simulink model "GFL_phasejump"  (R2022a)
settings: Solver=FixedStepAuto  StartTime=0.0  StopTime=t_end+t_sim_start  FixedStep=Ts  RelTol=1e-3
undefined symbols (not defined in the file or in its folder): Cf, dc_ref, DiscIntNeverNeededParam, dt, Id0, Id_limit, initial, Iq0, ki_pll, ki_v_dc, kp_pll, kp_v_dc, Lc, Lf, Lg1, Lg11, Lgg, m_v, phasejum, Rf, Rg1, Rg11, Rgg, Sbase, t0, t0_jump, t_sim_start, tc, Ts, v_sag, Vac_ref, Vbase, Vdc_ref, w_i_GFL, w_limit, w_pll, w_tau, w_tvc, Wbase, Y_dc, Zbase
libraries: spsVoltageMeasurementLib x41, spsCurrentMeasurementLib x36, spsThreePhaseSeriesRLCBranchLib x14, spsControlledVoltageSourceLib x12, spsSeriesRLCBranchLib x8, spsControlledCurrentSourceLib x4, spsIdealSwitchLib x3, spsThreePhaseBreakerLib x2, spsDCVoltageSourceLib x1, spsThreePhaseParallelRLCBranchLib x1, spsThreePhaseFaultLib x1, spspowerguiLib x1
(part 3 of 3)

== system GFL_phasejump/Grid-Following Inverter (Simulink Block)1/PLL (vabc -> vq)/Discrete PI ==
  note: Digital PI controller
      |
      | Author(s): Yitong Li
  enable : Inport
  reference : Inport  Port=2
  initial : Inport  Port=3
  actual : Inport  Port=4
  Discrete-Time Integrator : DiscreteIntegrator  gainval=1  ExternalReset=rising  InitialConditionSource=external  InitialCondition=initial  SampleTime=Ts  LimitOutput=on  UpperSaturationLimit=xmax  LowerSaturationLimit=xmin  ICPrevOutput=DiscIntNeverNeededParam  ICPrevScaledInput=DiscIntNeverNeededParam
  Ierror : Sum  Inputs=+-
  Ki : Gain  Gain=Ki  SaturateOnIntegerOverflow=on  OutDataTypeStr=Inherit: Same as input  ParamDataTypeStr=Inherit: Same as input
  Kp : Gain  Gain=Kp  SaturateOnIntegerOverflow=on  OutDataTypeStr=Inherit: Same as input  ParamDataTypeStr=Inherit: Same as input
  Perror : Sum  Inputs=-+
  Product : Product  RndMeth=Zero
  Product1 : Product  RndMeth=Zero
  Saturation : Saturate  UpperLimit=xmax  LowerLimit=xmin
  Scope : Scope  NumInputPorts=4
  Sum1 : Sum  SaturateOnIntegerOverflow=on
  Out : Outport
  wires:
  Product1/1 -> Ki/1
  Ierror/1 -> Product1/1
  Product/1 -> Kp/1
  Perror/1 -> Product/1
  actual/1 -> Perror/1, Ierror/2
  reference/1 -> Ierror/1, Perror/2
  initial/1 -> Discrete-Time Integrator/3
  enable/1 -> Product1/2, Product/2, Discrete-Time Integrator/2
  Discrete-Time Integrator/1 -> Scope/2, Sum1/2
  Kp/1 -> Scope/1, Sum1/1
  Ki/1 -> Discrete-Time Integrator/1
  Sum1/1 -> Saturation/1
  Saturation/1 -> Out/1

== system GFL_phasejump/Grid-Following Inverter (Simulink Block)1/PLL (vabc -> vq)/abc -> dq (Power-Invariant) ==
  note: Frame transformation from abc to dq.
      |
      | Author(s): Yitong Li
      |
      | Notes:
      |
      | The transformation is power-invariant.
      |
      | theta is the angle that d axis leads a axis.
      |
      | q axis leads d axis by 90 degrees.
  abc : Inport
  theta : Inport  Port=2
  ->d : Fcn  Expr=cos(u(4))*u(1) + cos(u(4)-2/3*pi)*u(2) + cos(u(4)-4/3*pi)*u(3)
  ->q : Fcn  Expr=-sin(u(4))*u(1) - sin(u(4)-2/3*pi)*u(2) - sin(u(4)-4/3*pi)*u(3)
  Gain : Gain  Gain=sqrt(2/3)
  Mux5 : Mux  Inputs=2
  Mux6 : Mux  Inputs=2
  dq : Outport
  wires:
  abc/1 -> Gain/1
  ->d/1 -> Mux6/1
  Gain/1 -> Mux5/1
  theta/1 -> Mux5/2
  ->q/1 -> Mux6/2
  Mux6/1 -> dq/1
  Mux5/1 -> ->d/1, ->q/1

== system GFL_phasejump/Grid-Following Inverter (Simulink Block)1/Voltage Controller/PI-DT-Estimated q ==
  actual : Inport
  initial : Inport  Port=2
  reference : Inport  Port=3
  enable : Inport  Port=4
  Discrete-Time Integrator : DiscreteIntegrator  gainval=1  ExternalReset=rising  InitialCondition=1  SampleTime=Ts  LimitOutput=on  UpperSaturationLimit=xmax  LowerSaturationLimit=xmin  ICPrevOutput=DiscIntNeverNeededParam  ICPrevScaledInput=DiscIntNeverNeededParam
  Ierror : Sum  Inputs=+-
  Ki : Gain  Gain=Ki  SaturateOnIntegerOverflow=on  OutDataTypeStr=Inherit: Same as input  ParamDataTypeStr=Inherit: Same as input
  Kp : Gain  Gain=Kp  SaturateOnIntegerOverflow=on  OutDataTypeStr=Inherit: Same as input  ParamDataTypeStr=Inherit: Same as input
  Perror : Sum  Inputs=-+
  Product : Product  RndMeth=Zero
  Product1 : Product  RndMeth=Zero
  Saturation : Saturate  UpperLimit=xmax  LowerLimit=xmin
  Sum1 : Sum  SaturateOnIntegerOverflow=on
  Out : Outport
  wires:
  Product1/1 -> Ki/1
  Ierror/1 -> Product1/1
  Product/1 -> Kp/1
  Perror/1 -> Product/1
  enable/1 -> Product1/2, Product/2, Discrete-Time Integrator/2
  Discrete-Time Integrator/1 -> Sum1/2
  Kp/1 -> Sum1/1
  Ki/1 -> Discrete-Time Integrator/1
  Sum1/1 -> Saturation/1
  Saturation/1 -> Out/1
  actual/1 -> Ierror/1, Perror/2
  reference/1 -> Ierror/2, Perror/1

== system GFL_phasejump/Grid-Following Inverter (Simulink Block)2/Current Controller/PI-DT-Estimated d ==
  enable : Inport
  reference : Inport  Port=2
  initial : Inport  Port=3
  actual : Inport  Port=4
  Discrete-Time Integrator : DiscreteIntegrator  gainval=1  ExternalReset=rising  InitialConditionSource=external  InitialCondition=initial  SampleTime=Ts  LimitOutput=on  UpperSaturationLimit=xmax  LowerSaturationLimit=xmin  ICPrevOutput=DiscIntNeverNeededParam  ICPrevScaledInput=DiscIntNeverNeededParam
  Ierror : Sum  Inputs=+-
  Ki : Gain  Gain=Ki  SaturateOnIntegerOverflow=on  OutDataTypeStr=Inherit: Same as input  ParamDataTypeStr=Inherit: Same as input
  Kp : Gain  Gain=Kp  SaturateOnIntegerOverflow=on  OutDataTypeStr=Inherit: Same as input  ParamDataTypeStr=Inherit: Same as input
  Perror : Sum  Inputs=-+
  Product : Product  RndMeth=Zero
  Product1 : Product  RndMeth=Zero
  Saturation : Saturate  UpperLimit=xmax  LowerLimit=xmin
  Sum1 : Sum  SaturateOnIntegerOverflow=on
  Out : Outport
  wires:
  Product1/1 -> Ki/1
  Ierror/1 -> Product1/1
  Product/1 -> Kp/1
  Perror/1 -> Product/1
  reference/1 -> Ierror/1, Perror/2
  actual/1 -> Ierror/2, Perror/1
  initial/1 -> Discrete-Time Integrator/3
  enable/1 -> Product1/2, Product/2, Discrete-Time Integrator/2
  Discrete-Time Integrator/1 -> Sum1/2
  Kp/1 -> Sum1/1
  Ki/1 -> Discrete-Time Integrator/1
  Sum1/1 -> Saturation/1
  Saturation/1 -> Out/1

== system GFL_phasejump/Grid-Following Inverter (Simulink Block)2/Current Controller/PI-DT-Estimated q ==
  actual : Inport
  initial : Inport  Port=2
  reference : Inport  Port=3
  enable : Inport  Port=4
  Discrete-Time Integrator : DiscreteIntegrator  gainval=1  ExternalReset=rising  InitialConditionSource=external  InitialCondition=initial  SampleTime=Ts  LimitOutput=on  UpperSaturationLimit=xmax  LowerSaturationLimit=xmin  ICPrevOutput=DiscIntNeverNeededParam  ICPrevScaledInput=DiscIntNeverNeededParam
  Ierror : Sum  Inputs=+-
  Ki : Gain  Gain=Ki  SaturateOnIntegerOverflow=on  OutDataTypeStr=Inherit: Same as input  ParamDataTypeStr=Inherit: Same as input
  Kp : Gain  Gain=Kp  SaturateOnIntegerOverflow=on  OutDataTypeStr=Inherit: Same as input  ParamDataTypeStr=Inherit: Same as input
  Perror : Sum  Inputs=-+
  Product : Product  RndMeth=Zero
  Product1 : Product  RndMeth=Zero
  Saturation : Saturate  UpperLimit=xmax  LowerLimit=xmin
  Sum1 : Sum  SaturateOnIntegerOverflow=on
  Out : Outport
  wires:
  Product1/1 -> Ki/1
  Ierror/1 -> Product1/1
  Product/1 -> Kp/1
  Perror/1 -> Product/1
  reference/1 -> Ierror/1, Perror/2
  actual/1 -> Perror/1, Ierror/2
  initial/1 -> Discrete-Time Integrator/3
  enable/1 -> Product1/2, Product/2, Discrete-Time Integrator/2
  Discrete-Time Integrator/1 -> Sum1/2
  Kp/1 -> Sum1/1
  Ki/1 -> Discrete-Time Integrator/1
  Sum1/1 -> Saturation/1
  Saturation/1 -> Out/1

== system GFL_phasejump/Grid-Following Inverter (Simulink Block)2/LCL Filter/LL -> LN1 ==
  note: Transformation from line-to-line voltage to line-to-neutral voltage.
      |
      | Author(s): Yitong Li
  In1 : Inport
  Fcn : Fcn  Expr=u[1]-u[3]
  Fcn1 : Fcn  Expr=u[2]-u[1]
  Fcn2 : Fcn  Expr=u[3]-u[2]
  Gain : Gain  Gain=1/3
  Mux9 : Mux  Inputs=3
  Out1 : Outport
  wires:
  In1/1 -> Gain/1
  Gain/1 -> Fcn/1, Fcn1/1, Fcn2/1
  Mux9/1 -> Out1/1
  Fcn2/1 -> Mux9/3
  Fcn1/1 -> Mux9/2
  Fcn/1 -> Mux9/1

== system GFL_phasejump/Grid-Following Inverter (Simulink Block)2/LCL Filter/LL -> LN2 ==
  note: Transformation from line-to-line voltage to line-to-neutral voltage.
      |
      | Author(s): Yitong Li
  In1 : Inport
  Fcn : Fcn  Expr=u[1]-u[3]
  Fcn1 : Fcn  Expr=u[2]-u[1]
  Fcn2 : Fcn  Expr=u[3]-u[2]
  Gain : Gain  Gain=1/3
  Mux9 : Mux  Inputs=3
  Out1 : Outport
  wires:
  In1/1 -> Gain/1
  Gain/1 -> Fcn/1, Fcn1/1, Fcn2/1
  Mux9/1 -> Out1/1
  Fcn2/1 -> Mux9/3
  Fcn1/1 -> Mux9/2
  Fcn/1 -> Mux9/1

== system GFL_phasejump/Grid-Following Inverter (Simulink Block)2/LCL Filter1/LL -> LN1 ==
  note: Transformation from line-to-line voltage to line-to-neutral voltage.
      |
      | Author(s): Yitong Li
  In1 : Inport
  Fcn : Fcn  Expr=u[1]-u[3]
  Fcn1 : Fcn  Expr=u[2]-u[1]
  Fcn2 : Fcn  Expr=u[3]-u[2]
  Gain : Gain  Gain=1/3
  Mux9 : Mux  Inputs=3
  Out1 : Outport
  wires:
  In1/1 -> Gain/1
  Gain/1 -> Fcn/1, Fcn1/1, Fcn2/1
  Mux9/1 -> Out1/1
  Fcn2/1 -> Mux9/3
  Fcn1/1 -> Mux9/2
  Fcn/1 -> Mux9/1

== system GFL_phasejump/Grid-Following Inverter (Simulink Block)2/LCL Filter1/LL -> LN2 ==
  note: Transformation from line-to-line voltage to line-to-neutral voltage.
      |
      | Author(s): Yitong Li
  In1 : Inport
  Fcn : Fcn  Expr=u[1]-u[3]
  Fcn1 : Fcn  Expr=u[2]-u[1]
  Fcn2 : Fcn  Expr=u[3]-u[2]
  Gain : Gain  Gain=1/3
  Mux9 : Mux  Inputs=3
  Out1 : Outport
  wires:
  In1/1 -> Gain/1
  Gain/1 -> Fcn/1, Fcn1/1, Fcn2/1
  Mux9/1 -> Out1/1
  Fcn2/1 -> Mux9/3
  Fcn1/1 -> Mux9/2
  Fcn/1 -> Mux9/1

== system GFL_phasejump/Grid-Following Inverter (Simulink Block)2/PLL (vabc -> vq)/Discrete PI ==
  note: Digital PI controller
      |
      | Author(s): Yitong Li
  enable : Inport
  reference : Inport  Port=2
  initial : Inport  Port=3
  actual : Inport  Port=4
  Discrete-Time Integrator : DiscreteIntegrator  gainval=1  ExternalReset=rising  InitialConditionSource=external  InitialCondition=initial  SampleTime=Ts  LimitOutput=on  UpperSaturationLimit=xmax  LowerSaturationLimit=xmin  ICPrevOutput=DiscIntNeverNeededParam  ICPrevScaledInput=DiscIntNeverNeededParam
  Ierror : Sum  Inputs=+-
  Ki : Gain  Gain=Ki  SaturateOnIntegerOverflow=on  OutDataTypeStr=Inherit: Same as input  ParamDataTypeStr=Inherit: Same as input
  Kp : Gain  Gain=Kp  SaturateOnIntegerOverflow=on  OutDataTypeStr=Inherit: Same as input  ParamDataTypeStr=Inherit: Same as input
  Perror : Sum  Inputs=-+
  Product : Product  RndMeth=Zero
  Product1 : Product  RndMeth=Zero
  Saturation : Saturate  UpperLimit=xmax  LowerLimit=xmin
  Scope : Scope  NumInputPorts=4
  Sum : Sum  Inputs=|+-
  Sum1 : Sum  SaturateOnIntegerOverflow=on
  pulse : Subsystem  AncestorBlock=SimplusGT/Single Pulse  mask{t0=t_sim_start-2}
      mask prompts: t0 "t0 (s), starting time"
  Out : Outport
  tag scope: Xint1IBR=global
  wires:
  Product1/1 -> Ki/1
  Ierror/1 -> Product1/1
  Product/1 -> Kp/1
  Perror/1 -> Product/1
  actual/1 -> Perror/1, Ierror/2
  reference/1 -> Ierror/1, Perror/2
  enable/1 -> Sum/1, Product1/2, Product/2
  Discrete-Time Integrator/1 -> Scope/2, Sum1/2, [Xint1IBR]
  Kp/1 -> Scope/1, Sum1/1
  Ki/1 -> Discrete-Time Integrator/1
  Sum1/1 -> Saturation/1
  Saturation/1 -> Out/1
  Sum/1 -> Scope/3, Discrete-Time Integrator/2
  initial/1 -> Discrete-Time Integrator/3
  pulse/1(Out) -> Sum/2

== system GFL_phasejump/Grid-Following Inverter (Simulink Block)2/PLL (vabc -> vq)/abc -> dq (Power-Invariant) ==
  note: Frame transformation from abc to dq.
      |
      | Author(s): Yitong Li
      |
      | Notes:
      |
      | The transformation is power-invariant.
      |
      | theta is the angle that d axis leads a axis.
      |
      | q axis leads d axis by 90 degrees.
  abc : Inport
  theta : Inport  Port=2
  ->d : Fcn  Expr=cos(u(4))*u(1) + cos(u(4)-2/3*pi)*u(2) + cos(u(4)-4/3*pi)*u(3)
  ->q : Fcn  Expr=-sin(u(4))*u(1) - sin(u(4)-2/3*pi)*u(2) - sin(u(4)-4/3*pi)*u(3)
  Gain : Gain  Gain=sqrt(2/3)
  Mux5 : Mux  Inputs=2
  Mux6 : Mux  Inputs=2
  dq : Outport
  wires:
  abc/1 -> Gain/1
  ->d/1 -> Mux6/1
  Gain/1 -> Mux5/1
  theta/1 -> Mux5/2
  ->q/1 -> Mux6/2
  Mux6/1 -> dq/1
  Mux5/1 -> ->d/1, ->q/1

== system GFL_phasejump/Grid-Following Inverter (Simulink Block)2/Voltage Controller/PI-DT-Estimated q ==
  actual : Inport
  initial : Inport  Port=2
  reference : Inport  Port=3
  enable : Inport  Port=4
  Discrete-Time Integrator : DiscreteIntegrator  gainval=1  ExternalReset=rising  InitialConditionSource=external  InitialCondition=1  SampleTime=Ts  LimitOutput=on  UpperSaturationLimit=xmax  LowerSaturationLimit=xmin  ICPrevOutput=DiscIntNeverNeededParam  ICPrevScaledInput=DiscIntNeverNeededParam
  Ierror : Sum  Inputs=+-
  Ki : Gain  Gain=Ki  SaturateOnIntegerOverflow=on  OutDataTypeStr=Inherit: Same as input  ParamDataTypeStr=Inherit: Same as input
  Kp : Gain  Gain=Kp  SaturateOnIntegerOverflow=on  OutDataTypeStr=Inherit: Same as input  ParamDataTypeStr=Inherit: Same as input
  Perror : Sum  Inputs=-+
  Product : Product  RndMeth=Zero
  Product1 : Product  RndMeth=Zero
  Saturation : Saturate  UpperLimit=xmax  LowerLimit=xmin
  Sum : Sum  Inputs=|+-
  Sum1 : Sum  SaturateOnIntegerOverflow=on
  pulse : Subsystem  AncestorBlock=SimplusGT/Single Pulse  mask{t0=t_sim_start-2}
      mask prompts: t0 "t0 (s), starting time"
  Out : Outport
  tag scope: Xint2IBR=global
  wires:
  Product1/1 -> Ki/1
  Ierror/1 -> Product1/1
  Product/1 -> Kp/1
  Perror/1 -> Product/1
  enable/1 -> Product/2, Product1/2, Sum/1
  Discrete-Time Integrator/1 -> [Xint2IBR], Sum1/2
  Kp/1 -> Sum1/1
  Ki/1 -> Discrete-Time Integrator/1
  Sum1/1 -> Saturation/1
  Saturation/1 -> Out/1
  actual/1 -> Ierror/1, Perror/2
  reference/1 -> Perror/1, Ierror/2
  initial/1 -> Discrete-Time Integrator/3
  pulse/1(Out) -> Sum/2
  Sum/1 -> Discrete-Time Integrator/2

== system GFL_phasejump/Grid-Following Inverter (Simulink Block)2/PLL (vabc -> vq)/Discrete PI/pulse ==
  note: Pulse generator
      |
      | Author(s): Yitong Li
  Product : Product
  Step : Step  Time=t0-0.01  SampleTime=0
  Step1 : Step  Time=t0  Before=1  After=0  SampleTime=0
  Out : Outport
  wires:
  Step1/1 -> Product/2
  Step/1 -> Product/1
  Product/1 -> Out/1

== system GFL_phasejump/Grid-Following Inverter (Simulink Block)2/Voltage Controller/PI-DT-Estimated q/pulse ==
  note: Pulse generator
      |
      | Author(s): Yitong Li
  Product : Product
  Step : Step  Time=t0-0.01  SampleTime=0
  Step1 : Step  Time=t0  Before=1  After=0  SampleTime=0
  Out : Outport
  wires:
  Step1/1 -> Product/2
  Step/1 -> Product/1
  Product/1 -> Out/1
